simulink model "RLS_PT1_debug"  (R2020a)
settings: Solver=FixedStepAuto  StartTime=0.0  StopTime=15  FixedStep=0.1  RelTol=1e-3
PostLoadFcn:
  | OPCua_RLS_PT1([], 'init', true);
StopFcn:
  | OPCua_RLS_PT1([], 'reset', true);
libraries: sldrtlib x1
CloseFcn:
  | OPCua_RLS_PT1([], 'finish', true);
settings Model: SimulationMode=accelerator  Creator=User  LastModifiedBy=User
settings SolverCC: ConcurrentTasks=on
settings DataIOCC: SaveOutput=off  SignalLogging=off  DSMLogging=off  SaveTime=off  ReturnWorkspaceOutputs=off
settings HardwareCC: ProdHWDeviceType=AMD->x86-64 (Windows64)
settings RTWCC: Description=Generic Real-Time Target  RTWCompilerOptimization=on
settings CodeAppCC: MaxIdLength=95

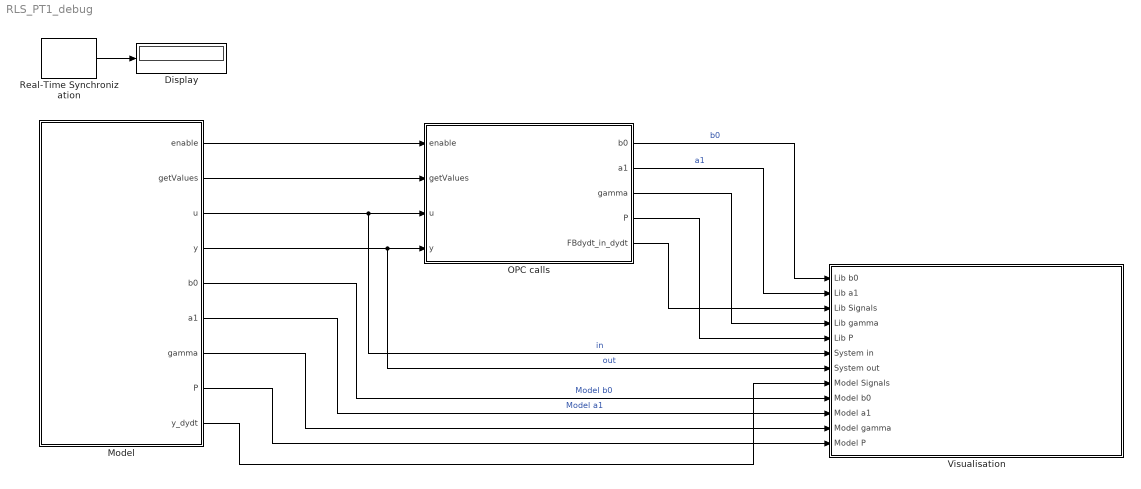
== system RLS_PT1_debug ==
  Display : Display
  Model : Subsystem  TreatAsAtomicUnit=on
  OPC calls : Subsystem  TreatAsAtomicUnit=on
  Real-Time Synchronization : sldrtlib/Real-Time Synchronization  SampleTime=0.1  MaxMissedTicks=Inf  ShowMissedTicks=on  YieldWhenWaiting=off
  Visualisation : Subsystem  TreatAsAtomicUnit=on
  wires:
  Model/1(enable) -> OPC calls/1(enable)
  Model/3(u) -> Visualisation/6(System in), OPC calls/3(u)  "in"
  Model/4(y) -> OPC calls/4(y), Visualisation/7(System out)  "out"
  Model/2(getValues) -> OPC calls/2(getValues)
  Real-Time Synchronization/1 -> Display/1
  OPC calls/1(b0) -> Visualisation/1(Lib b0)  "b0"
  OPC calls/2(a1) -> Visualisation/2(Lib a1)  "a1"
  OPC calls/3(gamma) -> Visualisation/4(Lib gamma)
  OPC calls/4(P) -> Visualisation/5(Lib P)
  OPC calls/5(FBdydt_in_dydt) -> Visualisation/3(Lib Signals)
  Model/5(b0) -> Visualisation/9(Model b0)  "Model b0"
  Model/6(a1) -> Visualisation/10(Model a1)  "Model a1"
  Model/7(gamma) -> Visualisation/11(Model gamma)
  Model/8(P) -> Visualisation/12(Model P)
  Model/9(y_dydt) -> Visualisation/8(Model Signals)

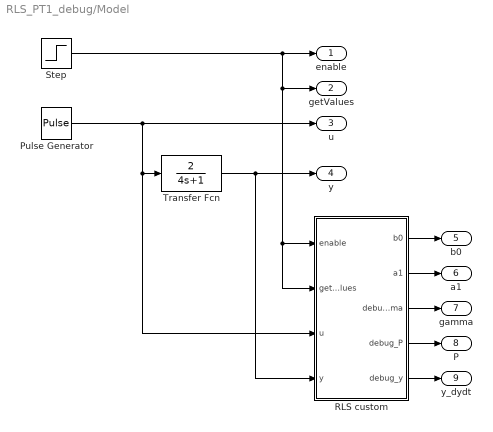
== system RLS_PT1_debug/Model ==
  Pulse Generator : DiscretePulseGenerator  PulseType=Time based  Period=10  PulseWidth=50
  RLS custom : MATLAB Function  TreatAsAtomicUnit=on
  Step : Step  SampleTime=0
  Transfer Fcn : TransferFcn  Numerator=[2]  Denominator=[4 1]
  enable : Outport
  getValues : Outport  Port=2
  u : Outport  Port=3
  y : Outport  Port=4
  b0 : Outport  Port=5
  a1 : Outport  Port=6
  gamma : Outport  Port=7
  P : Outport  Port=8
  y_dydt : Outport  Port=9
  wires:
  Pulse Generator/1 -> Transfer Fcn/1, RLS custom/3(u), u/1
  Step/1 -> getValues/1, RLS custom/2(getValues), RLS custom/1(enable), enable/1
  Transfer Fcn/1 -> y/1, RLS custom/4(y)
  RLS custom/1(b0) -> b0/1
  RLS custom/2(a1) -> a1/1
  RLS custom/3(debug_gamma) -> gamma/1
  RLS custom/4(debug_P) -> P/1
  RLS custom/5(debug_y) -> y_dydt/1

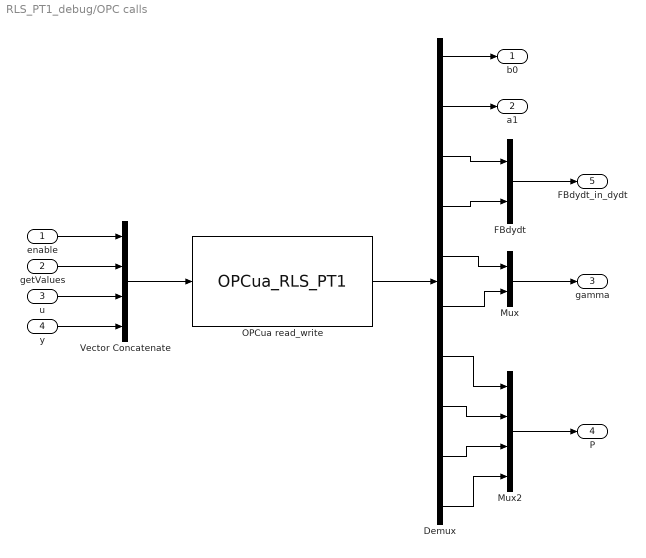
== system RLS_PT1_debug/OPC calls ==
  enable : Inport
  getValues : Inport  Port=2
  u : Inport  Port=3
  y : Inport  Port=4
  Demux : Demux  Outputs=10
  FBdydt : Mux  Inputs=2
  Mux : Mux  Inputs=2
  Mux2 : Mux
  OPCua read_write : MATLABFcn  MATLABFcn=OPCua_RLS_PT1  OutputDimensions=10
  Vector Concatenate : Concatenate  NumInputs=4
  b0 : Outport
  a1 : Outport  Port=2
  gamma : Outport  Port=3
  P : Outport  Port=4
  FBdydt_in_dydt : Outport  Port=5
  wires:
  Demux/1 -> b0/1
  enable/1 -> Vector Concatenate/1
  Demux/2 -> a1/1
  u/1 -> Vector Concatenate/3
  y/1 -> Vector Concatenate/4
  Vector Concatenate/1 -> OPCua read_write/1
  OPCua read_write/1 -> Demux/1
  getValues/1 -> Vector Concatenate/2
  Demux/4 -> FBdydt/2
  Demux/3 -> FBdydt/1
  FBdydt/1 -> FBdydt_in_dydt/1
  Mux/1 -> gamma/1
  Mux2/1 -> P/1
  Demux/10 -> Mux2/4
  Demux/5 -> Mux/1
  Demux/6 -> Mux/2
  Demux/7 -> Mux2/1
  Demux/8 -> Mux2/2
  Demux/9 -> Mux2/3

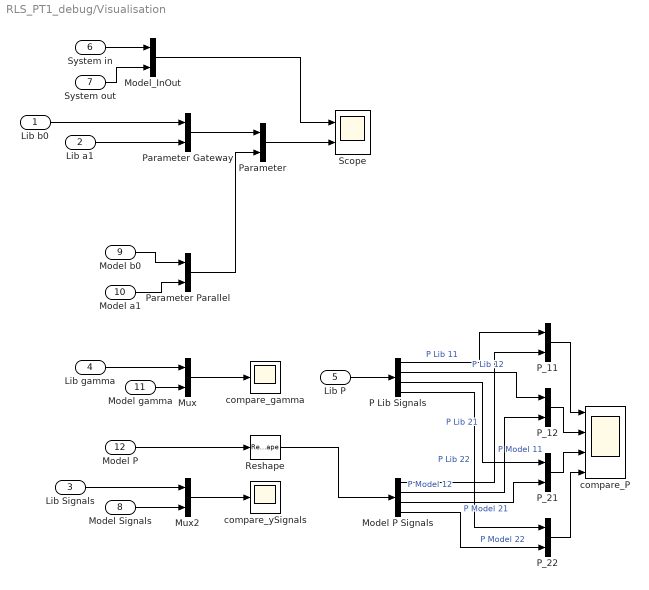
== system RLS_PT1_debug/Visualisation ==
  Lib b0 : Inport
  Lib a1 : Inport  Port=2
  Lib Signals : Inport  Port=3
  Lib gamma : Inport  Port=4
  Lib P : Inport  Port=5
  System in : Inport  Port=6
  System out : Inport  Port=7
  Model Signals : Inport  Port=8
  Model b0 : Inport  Port=9
  Model a1 : Inport  Port=10
  Model gamma : Inport  Port=11
  Model P : Inport  Port=12
  Model P Signals : Demux
  Model_InOut : Mux  Inputs=2
  Mux : Mux  Inputs=2
  Mux2 : Mux  Inputs=2
  P Lib Signals : Demux
  P_{11..12,21..22} (4 alike) : Mux  Inputs=2
  Parameter : Mux  Inputs=2
  Parameter Gateway : Mux  Inputs=2
  Parameter Parallel : Mux  Inputs=2
  Reshape : Reshape
  Scope : Scope  NumInputPorts=2
  compare_P : Scope  NumInputPorts=4
  compare_gamma : Scope
  compare_ySignals : Scope
  wires:
  Model P Signals/3 -> P_21/2  "P Model 21"
  Parameter/1 -> Scope/2
  Model a1/1 -> Parameter Parallel/2
  Lib gamma/1 -> Mux/1
  Mux2/1 -> compare_ySignals/1
  Model Signals/1 -> Mux2/2
  Lib P/1 -> P Lib Signals/1
  Mux/1 -> compare_gamma/1
  Model_InOut/1 -> Scope/1
  Model P Signals/2 -> P_12/2  "P Model 12"
  P_12/1 -> compare_P/2
  Parameter Gateway/1 -> Parameter/1
  P Lib Signals/1 -> P_11/1  "P Lib 11"
  Model P/1 -> Reshape/1
  Reshape/1 -> Model P Signals/1
  P Lib Signals/2 -> P_12/1  "P Lib 12"
  P Lib Signals/4 -> P_22/1  "P Lib 22"
  Model P Signals/1 -> P_11/2  "P Model 11"
  Model P Signals/4 -> P_22/2  "P Model 22"
  Parameter Parallel/1 -> Parameter/2
  P_22/1 -> compare_P/4
  P_11/1 -> compare_P/1
  P Lib Signals/3 -> P_21/1  "P Lib 21"
  P_21/1 -> compare_P/3
  Model b0/1 -> Parameter Parallel/1
  System out/1 -> Model_InOut/2
  Lib Signals/1 -> Mux2/1
  System in/1 -> Model_InOut/1
  Model gamma/1 -> Mux/2
  Lib b0/1 -> Parameter Gateway/1
  Lib a1/1 -> Parameter Gateway/2

== matlab function RLS_PT1_debug/Model/RLS custom ==
  settings: updateMethod=DISCRETE
  data: enable input; getValues input; u input; b0 output; y input; a1 output; debug_gamma output; debug_P output; debug_y output
function [b0, a1, debug_gamma, debug_P, debug_y] = fcn(enable, getValues, u, y)
% RLS implementation simulating the gateway solution as close as poissible
    % RLS Parameters
    lambda = 0.9; % forgetting factor
    P0 = 1.0e6; % initial value of P diagonal
    dt = 0.1; % step size in s
        
    % keep state of RLS
    persistent P Theta ylast init
    
    if isempty(init)
        init = 1;
    end
    
    if isempty(ylast)
        ylast = 0.0;
    end
    
    if isempty(P)
        P = [[P0 0]; [0 P0]];
    end
    
    if isempty(Theta)
        Theta = [0; 0];
    end

    debug_gamma = [0; 0];
    debug_P = [[0 0]; [0 0]];
    debug_y = [0 0];
    
    if enable
        if init
            P = [[P0 0]; [0 P0]];
            Theta = [0; 0];
            init = 0;
        end
        % create necessary inputs / variables
        dydt = (y-ylast)/dt;
        x = [u; -dydt];
        xT = transpose(x);
        % RLS calculation
        gamma = (P*x) / (lambda + xT*P*x);
        Theta = Theta + gamma*(y - xT*Theta);
        P = (P - gamma*xT*P)/lambda;
        
        debug_gamma = gamma;
        debug_P = P;
        debug_y = [y dydt];
    else
        init = 1;
    end
    
    if getValues
        b0 = Theta(1);
        a1 = Theta(2);
    else
        b0 = 0;
        a1 = 0;
    end
    
    % keep track on ylast in every case
    ylast = y;
end
